simulink model "GenOptRockerMomtryDisHndlr_BSWModel"  (R2017b)
settings: configuration reference "JD_ConfigsetAUTOSARMulti10msec" (kept outside this file)
libraries: AUTOSAR_BSW_ClientServerLibrary x1
settings Model: Creator=KIH3CPW  LastModifiedBy=KIH3CPW
settings ConfigSetRef: SourceLocation=Base Workspace

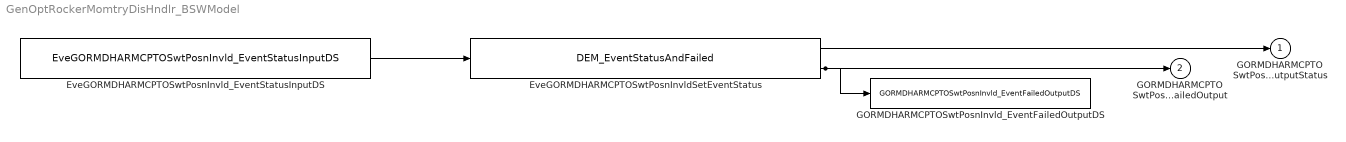
== system GenOptRockerMomtryDisHndlr_BSWModel ==
  EveGORMDHARMCPTOSwtPosnInvldSetEventStatus : AUTOSAR_BSW_ClientServerLibrary/DEM_EventStatusAndFailed  Units=seconds  FaultSetTime=FaultSetTime
  EveGORMDHARMCPTOSwtPosnInvld_EventStatusInputDS : DataStoreRead  DataStoreName=EveGORMDHARMCPTOSwtPosnInvld_EventStatusInputDS
  GORMDHARMCPTOSwtPosnInvld_EventFailedOutputDS : DataStoreWrite  DataStoreName=GORMDHARMCPTOSwtPosnInvld_EventFailedOutputDS
  GORMDHARMCPTOSwtPosnInvldOutputStatus : Outport
  GORMDHARMCPTOSwtPosnInvldFailedOutput : Outport  Port=2
  wires:
  EveGORMDHARMCPTOSwtPosnInvld_EventStatusInputDS/1 -> EveGORMDHARMCPTOSwtPosnInvldSetEventStatus/1
  EveGORMDHARMCPTOSwtPosnInvldSetEventStatus/1 -> GORMDHARMCPTOSwtPosnInvldOutputStatus/1
  EveGORMDHARMCPTOSwtPosnInvldSetEventStatus/2 -> GORMDHARMCPTOSwtPosnInvldFailedOutput/1, GORMDHARMCPTOSwtPosnInvld_EventFailedOutputDS/1
